simulink model "HammingEncoder"  (R2020b)
settings: Solver=VariableStepAuto  StartTime=0.0  StopTime=10.0  RelTol=1e-3
settings Model: Creator=12643  LastModifiedBy=12643

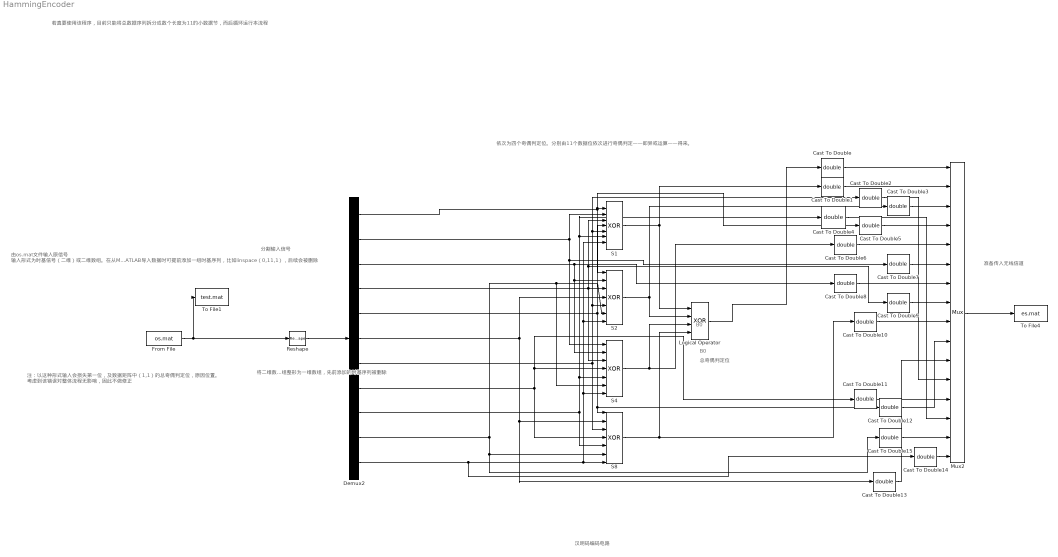
== system HammingEncoder ==
  note: B0
  note: B0
  note: 依次为四个奇偶判定位。分别由11个数据位依次进行奇偶判定——即异或运算——得来。
  note: 汉明码编码电路
  note: 由os.mat文件输入原信号
      | 输入形式为时基信号（二维）或二维数组。在从MATLAB导入数据时可提前添加一组时基序列，比如linspace（0,11,1），后续会被删除
  note: 将二维数组整形为一维数组，先前添加的时基序列被删除
  note: 分割输入信号
  note: 注：以这种形式输入会损失第一位，及数据矩阵中（1,1）的总奇偶判定位，原因位置。
      | 考虑到该错误对整体流程无影响，因此不做修正
  note: 若真要使用该程序，目前只能将总数据序列拆分成数个长度为11的小数据节，而后循环运行本流程
  note: 总奇偶判定位
  note: 准备传入无线信道
  Cast To Double{,1..15} (16 alike) : DataTypeConversion  OutDataTypeStr=double
  Demux2 : Demux  Outputs=11
  From File : FromFile  FileName=os.mat  SampleTime=0
  Logical Operator : Logic  Operator=XOR  Inputs=4  AllPortsSameDT=off  OutDataTypeStr=boolean
  Mux2 : Mux  Inputs=16
  Reshape : Reshape  OutputDimensionality=Customize  OutputDimensions=[11,1]
  S{1..2,4,8} (4 alike) : Logic  Operator=XOR  Inputs=7  AllPortsSameDT=off  OutDataTypeStr=boolean
  To File1 : ToFile  Filename=test.mat  MatrixName=test
  To File4 : ToFile  Filename=es.mat  MatrixName=es
  wires:
  Demux2/1 -> S1/1, Cast To Double5/1, S2/1
  Demux2/2 -> Cast To Double7/1, S4/1, S1/2
  Demux2/4 -> S1/3, Cast To Double9/1, S4/3, S2/3
  Demux2/5 -> S8/1, Cast To Double12/1, S1/4
  Demux2/7 -> Cast To Double2/1, S1/5, S2/5, S8/3
  Demux2/9 -> Cast To Double4/1, S1/6, S4/5, S8/5
  Demux2/11 -> S1/7, S2/7, S4/7, S8/7, Cast To Double14/1
  Demux2/3 -> Cast To Double8/1, S4/2, S2/2
  Demux2/6 -> Cast To Double13/1, S8/2, S2/4
  Demux2/10 -> Cast To Double15/1, S8/6, S2/6, S4/6
  Demux2/8 -> Cast To Double11/1, S4/4, S8/4
  S1/1 -> Cast To Double1/1, Logical Operator/1
  S2/1 -> Cast To Double3/1, Logical Operator/2
  S4/1 -> Cast To Double6/1, Logical Operator/3
  S8/1 -> Logical Operator/4, Cast To Double10/1
  From File/1 -> To File1/1, Reshape/1
  Reshape/1 -> Demux2/1
  Logical Operator/1 -> Cast To Double/1
  Mux2/1 -> To File4/1
  Cast To Double/1 -> Mux2/1
  Cast To Double1/1 -> Mux2/2
  Cast To Double2/1 -> Mux2/12
  Cast To Double3/1 -> Mux2/3
  Cast To Double4/1 -> Mux2/14
  Cast To Double5/1 -> Mux2/4
  Cast To Double6/1 -> Mux2/5
  Cast To Double7/1 -> Mux2/6
  Cast To Double8/1 -> Mux2/7
  Cast To Double9/1 -> Mux2/8
  Cast To Double10/1 -> Mux2/9
  Cast To Double11/1 -> Mux2/13
  Cast To Double12/1 -> Mux2/10
  Cast To Double13/1 -> Mux2/11
  Cast To Double14/1 -> Mux2/16
  Cast To Double15/1 -> Mux2/15
